simulink library "csu_lat_landing_approach_targeting_lib"  (R2015b)
settings: Solver=ode45  StartTime=0.0  StopTime=10.0  RelTol=1e-3
values from neighbouring files (symbols this model uses):
  gdn_targeting_lateral_accel_gain = [0.5  0.5]    [csu_lat_landing_approach_targeting_init.m]
  gdn_targeting_lateral_accel_limit = [2.0  2.0]    [csu_lat_landing_approach_targeting_init.m]
  gdn_targeting_velocity_error_gain = [1.8  1.8  2.0]    [csu_lat_landing_approach_targeting_init.m]
  gdn_targeting_velocity_error_limit = [10.0 10.0 30.0]    [csu_lat_landing_approach_targeting_init.m]
libraries: simulink x9, util_info_lib x1, util_common_lib x1
settings Model: Creator=escrane  LastModifiedBy=jimkaidy
settings DataIOCC: SaveFormat=Array
settings DebuggingCC: UnderspecifiedInitializationDetection=Classic  MergeDetectMultiDrivingBlocksExec=none  SolverPrmCheckMsg=warning
settings HardwareCC: ProdBitPerPointer=32  ProdLargestAtomicFloat=None  ProdIntDivRoundTo=Undefined  ProdEndianess=Unspecified  ProdWordSize=32  ProdHWDeviceType=32-bit Generic
settings GRTTargetCC: GeneratePreprocessorConditionals=Disable all
settings ConfigComp: CovModelRefEnable=Off  CovSFcnEnable=off

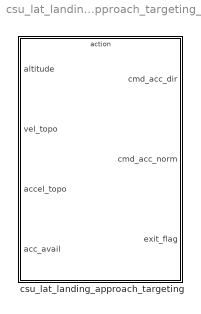
== system csu_lat_landing_approach_targeting_lib ==
  csu_lat_landing_approach_targeting : Subsystem  TreatAsAtomicUnit=on

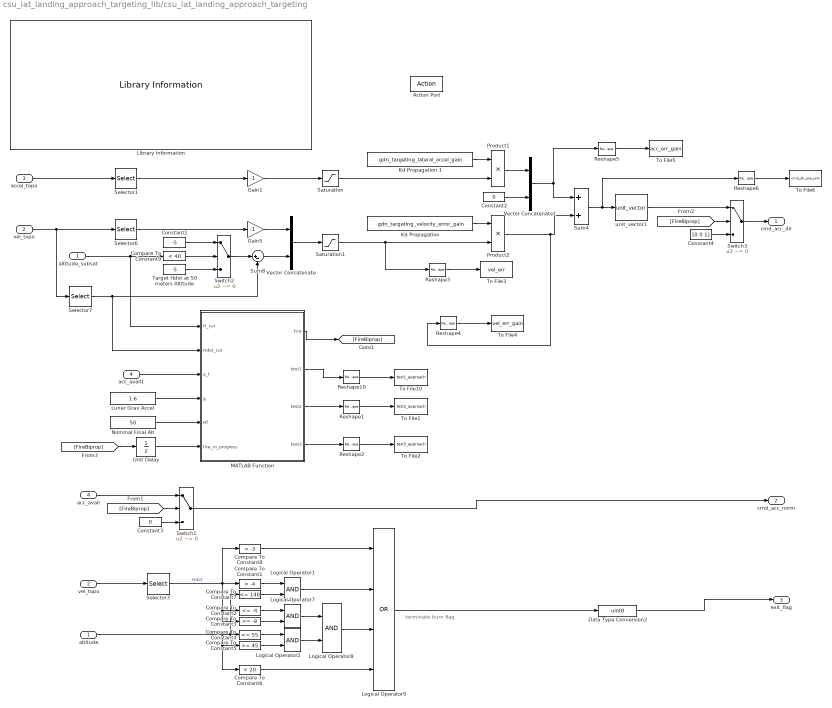
== system csu_lat_landing_approach_targeting_lib/csu_lat_landing_approach_targeting ==
  note: terminate burn flag
  "altitude " : Inport
  "vel_topo " : Inport  Port=2
  accel_topo : Inport  Port=3
  acc_avail : Inport  Port=4
  Action Port : ActionPort
  Compare To Constant1 : simulink/Logic and Bit Operations/Compare To Constant  relop=>  const=-4  OutDataTypeStr=boolean
  Compare To Constant2 : simulink/Logic and Bit Operations/Compare To Constant  relop=<=  const=-4  OutDataTypeStr=boolean
  Compare To Constant3 : simulink/Logic and Bit Operations/Compare To Constant  relop=>=  const=-8  OutDataTypeStr=boolean
  Compare To Constant4 : simulink/Logic and Bit Operations/Compare To Constant  relop=<=  const=55  OutDataTypeStr=boolean
  Compare To Constant5 : simulink/Logic and Bit Operations/Compare To Constant  relop=>=  const=45  OutDataTypeStr=boolean
  Compare To Constant6 : simulink/Logic and Bit Operations/Compare To Constant  relop=<  const=20  OutDataTypeStr=boolean
  Compare To Constant7 : simulink/Logic and Bit Operations/Compare To Constant  relop=<=  const=140  OutDataTypeStr=boolean
  Compare To Constant8 : simulink/Logic and Bit Operations/Compare To Constant  relop=>  const=-3  OutDataTypeStr=boolean
  Compare To Constant9 : simulink/Logic and Bit Operations/Compare To Constant  relop=<  const=40  OutDataTypeStr=boolean
  Constant1 : Constant  Value=-5
  Constant2 : Constant  Value=0
  Constant3 : Constant  Value=0
  Constant4 : Constant  Value=[0 0 1]
  Data Type Conversion2 : DataTypeConversion  OutDataTypeStr=uint8
  Gain1 : Gain  Gain=-1
  Gain5 : Gain  Gain=-1
  "Kd Propagation " : Constant  Value=gdn_targeting_velocity_error_gain
  Kd Propagation 1 : Constant  Value=gdn_targeting_lateral_accel_gain
  Library Information : util_info_lib/Library Information  owner='NONE'
  Logical Operator{1..2,7..8} (4 alike) : Logic  AllPortsSameDT=off  OutDataTypeStr=boolean
  Logical Operator9 : Logic  Operator=OR  Inputs=4  AllPortsSameDT=off  OutDataTypeStr=boolean
  Lunar Grav Accel : Constant  Value=1.6
  MATLAB Function : MATLAB Function  TreatAsAtomicUnit=on
  "Nominal Final Alt " : Constant  Value=50
  Product1 : Product
  Product2 : Product
  Reshape{1..6,10} (7 alike) : Reshape
  Saturation : Saturate  UpperLimit=gdn_targeting_lateral_accel_limit  LowerLimit=-gdn_targeting_lateral_accel_limit
  Saturation1 : Saturate  UpperLimit=gdn_targeting_velocity_error_limit  LowerLimit=-gdn_targeting_velocity_error_limit
  Selector1 : Selector  InputPortWidth=3  IndexOptions=Index vector (dialog)  Indices=[1 2]  OutputSizes=1
  Selector3 : Selector  InputPortWidth=3  IndexOptions=Index vector (dialog)  Indices=[3]  OutputSizes=1
  Selector6 : Selector  InputPortWidth=3  IndexOptions=Index vector (dialog)  Indices=[1 2]  OutputSizes=1
  Selector7 : Selector  InputPortWidth=3  IndexOptions=Index vector (dialog)  Indices=[3]  OutputSizes=1
  Sum4 : Sum
  Sum8 : Sum  Inputs=|+-
  Switch1 : Switch  Criteria=u2 ~= 0
  Switch2 : Switch  Criteria=u2 ~= 0
  Switch3 : Switch  Criteria=u2 ~= 0
  Target Hdot at 50 meters Altitude : Constant  Value=-5
  To File1 : ToFile  Filename=test2_approach  MatrixName=test2_approach  SaveFormat=Timeseries
  To File10 : ToFile  Filename=test1_approach  MatrixName=test1_approach  SaveFormat=Timeseries
  To File2 : ToFile  Filename=test3_approach  MatrixName=test3_approach  SaveFormat=Timeseries
  To File3 : ToFile  Filename=vel_err  MatrixName=vel_err  SaveFormat=Timeseries
  To File4 : ToFile  Filename=vel_err_gain  MatrixName=vel_err_gain  SaveFormat=Timeseries
  To File5 : ToFile  Filename=acc_err_gain  MatrixName=acc_err_gain  SaveFormat=Timeseries
  To File6 : ToFile  Filename=cmd_dir_pre_unit  MatrixName=cmd_dir_pre_unit  SaveFormat=Timeseries
  Unit Delay : UnitDelay  SampleTime=-1
  Vector Concatenate : Concatenate
  Vector Concatenate1 : Concatenate
  acc_avail1 : InportShadow  Port=4
  altitude_subsat : InportShadow
  unit_vector1 : util_common_lib/unit_vector  SystemSampleTime=-1
  vel_topo : InportShadow  Port=2
  cmd_acc_dir : Outport  InitialOutput=[0 0 1]'
  cmd_acc_norm : Outport  Port=2  InitialOutput=0
  exit_flag : Outport  Port=3  InitialOutput=0
  wires:
  Saturation/1 -> Product1/2
  Product1/1 -> Vector Concatenate1/1
  Constant2/1 -> Vector Concatenate1/2
  Product2/1 -> Reshape4/1, Sum4/2
  Vector Concatenate1/1 -> Sum4/1, Reshape5/1
  Gain1/1 -> Saturation/1
  Kd Propagation 1/1 -> Product1/1
  Selector1/1 -> Gain1/1
  accel_topo/1 -> Selector1/1
  Saturation1/1 -> Reshape3/1, Product2/2
  Sum8/1 -> Vector Concatenate/2
  Compare To Constant9/1 -> Switch2/2
  Constant1/1 -> Switch2/1
  Target Hdot at 50 meters Altitude/1 -> Switch2/3
  Logical Operator9/1 -> Data Type Conversion2/1
  Data Type Conversion2/1 -> exit_flag/1
  "vel_topo "/1 -> Selector7/1, Selector6/1
  Sum4/1 -> Reshape6/1, unit_vector1/1
  Compare To Constant3/1 -> Logical Operator7/2
  Compare To Constant6/1 -> Logical Operator9/4
  "altitude "/1 -> Compare To Constant7/1, Compare To Constant4/1, Compare To Constant5/1, Compare To Constant6/1
  Selector3/1 -> Compare To Constant8/1, Compare To Constant1/1, Compare To Constant2/1, Compare To Constant3/1  "Hdot"
  Compare To Constant2/1 -> Logical Operator7/1
  Logical Operator8/1 -> Logical Operator9/3
  vel_topo/1 -> Selector3/1
  MATLAB Function/1(Fire) -> [FireBiprop]
  Vector Concatenate/1 -> Saturation1/1
  Gain5/1 -> Vector Concatenate/1
  Selector7/1 -> MATLAB Function/2(Hdot_cur), Sum8/2
  Switch2/1 -> Sum8/1
  Selector6/1 -> Gain5/1
  "Kd Propagation "/1 -> Product2/1
  Switch1/1 -> cmd_acc_norm/1
  Constant3/1 -> Switch1/3
  [FireBiprop] -> Switch1/2
  Logical Operator7/1 -> Logical Operator8/1
  Logical Operator2/1 -> Logical Operator8/2
  acc_avail1/1 -> MATLAB Function/3(a_t)
  [FireBiprop] -> Unit Delay/1
  Unit Delay/1 -> MATLAB Function/6(fire_in_progress)
  "Nominal Final Alt "/1 -> MATLAB Function/5(Hf)
  Lunar Grav Accel/1 -> MATLAB Function/4(g)
  Compare To Constant4/1 -> Logical Operator2/1
  Compare To Constant5/1 -> Logical Operator2/2
  acc_avail/1 -> Switch1/1
  Compare To Constant1/1 -> Logical Operator1/1
  Compare To Constant7/1 -> Logical Operator1/2
  Logical Operator1/1 -> Logical Operator9/2
  Compare To Constant8/1 -> Logical Operator9/1
  altitude_subsat/1 -> Compare To Constant9/1, MATLAB Function/1(H_cur)
  MATLAB Function/2(test1) -> Reshape10/1
  MATLAB Function/3(test2) -> Reshape1/1
  MATLAB Function/4(test3) -> Reshape2/1
  Reshape10/1 -> To File10/1
  Reshape1/1 -> To File1/1
  Reshape2/1 -> To File2/1
  Reshape3/1 -> To File3/1
  Reshape4/1 -> To File4/1
  Reshape5/1 -> To File5/1
  Reshape6/1 -> To File6/1
  Constant4/1 -> Switch3/3
  [FireBiprop] -> Switch3/2
  unit_vector1/1 -> Switch3/1
  Switch3/1 -> cmd_acc_dir/1

== matlab function csu_lat_landing_approach_targeting_lib/csu_lat_landing_approach_targeting/MATLAB Function ==
  data: H_cur input; Hdot_cur input; Fire output boolean; a_t input; g input; Hf input; fire_in_progress input boolean; test1 output; test2 output; test3 output
function [Fire, test1, test2, test3] = ApproachTargeting(H_cur,Hdot_cur,a_t,g,Hf,fire_in_progress)
%#codegen

Hi = H_cur;
Hdoti = Hdot_cur;

if fire_in_progress == false
    
    if (Hdoti^2 - 2*(a_t - g)*(Hi - Hf)) >= 0 && Hdoti < 0
       tf = (-Hdoti + sqrt(Hdoti^2 - 2*(a_t - g)*(Hi - Hf)))/abs(a_t - g);
    else
      tf = -1;
    end

    if tf > 0; 
        Fire = true;
    else
        Fire = false;
    end
else   
    Fire = true;
end

test1 = (Hdoti^2 - 2*(a_t - g)*(Hi - Hf));

test2 = 2*(a_t - g)*(Hi - Hf);

test3 = (-Hdoti + sqrt(Hdoti^2 - 2*(a_t - g)*(Hi - Hf)))/abs(a_t - g);
